simulink library "SUB_L4_Task_10ms_SUB_BRKPEDARB"  (R2018a)
settings: Solver=VariableStepAuto  StartTime=0.0  StopTime=10.0  RelTol=1e-3
libraries: EmE_MBD_Blockset x73, PTC_MBDS_LIB x6, simulink x3
(part 2 of 2)

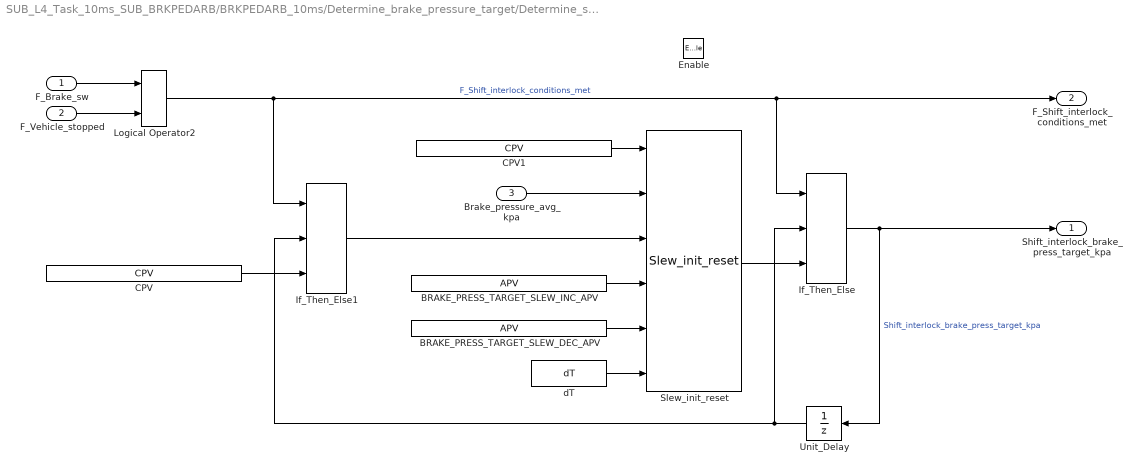
== system SUB_L4_Task_10ms_SUB_BRKPEDARB/BRKPEDARB_10ms/Determine_brake_pressure_target/Determine_shift_interlock_brake_pressure_target ==
  F_Brake_sw : Inport
  F_Vehicle_stopped : Inport  Port=2
  Brake_pressure_avg_kpa : Inport  Port=3
  Enable : EnablePort  StatesWhenEnabling=reset
      settings: AttributesFormatString=States when enabling: %<StatesWhenEnabling>
      settings: CopyFcn=|
      | try
      | L = find_system(get(gcbh,'Parent'),'BlockType','Outport');
      | M = find_system(get(gcbh,'Parent'),'BlockType','EnablePort');
      | N = find_system(get(gcbh,'Parent'),'BlockType','TriggerPort');
      | anyoutports = ~isempty(L);
      | anyenableports = ~isempty(M);
      | anytriggerports = ~isempty(N);
      | sys = get_param(L,'Handle');
      | noutports = length(sys);
      | if (anyoutports),
      | for i = 1:noutports,
      | set(sys{i},'AttributesFormatString','IC: %<InitialOutput>\nDisabled value: %<OutputWhenDisabled>')
      | end;
      | end;
      | catch
      | end;
      | clear i L M N anyoutports anyenableports anytriggerports sys noutports
      settings: DeleteFcn=|
      | try
      | L = find_system(get(gcbh,'Parent'),'BlockType','Outport');
      | M = find_system(get(gcbh,'Parent'),'BlockType','EnablePort');
      | N = find_system(get(gcbh,'Parent'),'BlockType','TriggerPort');
      | anyoutports = ~isempty(L);
      | anyenableports = ~isempty(M);
      | anytriggerports = ~isempty(N);
      | sys = get_param(L,'Handle');
      | noutports = length(sys);
      | if ((anyoutports) && (~anytriggerports)),
      | for i = 1:noutports,
      | set(sys{i},'AttributesFormatString','')
      | end;
      | end;
      | catch
      | end;
      | clear i L M N anyoutports anyenableports anytriggerports sys noutports
      settings: NameChangeFcn=|
      | try
      | L = find_system(get(gcbh,'Parent'),'BlockType','Outport');
      | M = find_system(get(gcbh,'Parent'),'BlockType','EnablePort');
      | N = find_system(get(gcbh,'Parent'),'BlockType','TriggerPort');
      | anyoutports = ~isempty(L);
      | anyenableports = ~isempty(M);
      | anytriggerports = ~isempty(N);
      | sys = get_param(L,'Handle');
      | noutports = length(sys);
      | if (anyoutports),
      | for i = 1:noutports,
      | set(sys{i},'AttributesFormatString','IC: %<InitialOutput>\nDisabled value: %<OutputWhenDisabled>')
      | end;
      | end;
      | catch
      | end
      | clear i L M N anyoutports anyenableports anytriggerports sys noutports
      settings: MoveFcn=|
      | try
      | L = find_system(get(gcbh,'Parent'),'BlockType','Outport');
      | M = find_system(get(gcbh,'Parent'),'BlockType','EnablePort');
      | N = find_system(get(gcbh,'Parent'),'BlockType','TriggerPort');
      | anyoutports = ~isempty(L);
      | anyenableports = ~isempty(M);
      | anytriggerports = ~isempty(N);
      | sys = get_param(L,'Handle');
      | noutports = length(sys);
      | if (anyoutports),
      | for i = 1:noutports,
      | set(sys{i},'AttributesFormatString','IC: %<InitialOutput>\nDisabled value: %<OutputWhenDisabled>')
      | end;
      | end;
      | catch
      | end;
      | clear i L M N anyoutports anyenableports anytriggerports sys noutports
  BRAKE_PRESS_TARGET_SLEW_DEC_APV : EmE_MBD_Blockset/Sources/APV  conval=5000
      settings: SourceProductName=PACCAR EmE MBD Blockset
  BRAKE_PRESS_TARGET_SLEW_INC_APV : EmE_MBD_Blockset/Sources/APV  conval=30
      settings: SourceProductName=PACCAR EmE MBD Blockset
  CPV : EmE_MBD_Blockset/Sources/CPV  conval=865
      settings: SourceProductName=PACCAR EmE MBD Blockset
  CPV1 : EmE_MBD_Blockset/Sources/CPV  conval=false
      settings: SourceProductName=PACCAR EmE MBD Blockset
  If_Then_Else : EmE_MBD_Blockset/Signal Routing/If_Then_Else
      settings: SourceProductName=PACCAR EmE MBD Blockset
  If_Then_Else1 : EmE_MBD_Blockset/Signal Routing/If_Then_Else
      settings: SourceProductName=PACCAR EmE MBD Blockset
  Logical Operator2 : EmE_MBD_Blockset/Logic and Bit Operations/Logical Operator  Operator=AND  Inputs=2
      settings: SourceProductName=PACCAR EmE MBD Blockset
  Slew_init_reset : EmE_MBD_Blockset/Math Operators/Slew_init_reset
      settings: SourceProductName=PACCAR EmE MBD Blockset
  Unit_Delay : UnitDelay  SampleTime=-1
      settings: AttributesFormatString=IC: %<vinit>
  dT : EmE_MBD_Blockset/Sources/dT
      settings: SourceProductName=PACCAR EmE MBD Blockset
  Shift_interlock_brake_press_target_kpa : Outport  OutputWhenDisabled=reset  InitialOutput=0
      settings: AttributesFormatString=IC: %<InitialOutput>\nDisabled value: %<OutputWhenDisabled>
  F_Shift_interlock_conditions_met : Outport  Port=2  OutputWhenDisabled=reset  InitialOutput=false
      settings: AttributesFormatString=IC: %<InitialOutput>\nDisabled value: %<OutputWhenDisabled>
  wires:
  CPV1/1 -> Slew_init_reset/1
  Brake_pressure_avg_kpa/1 -> Slew_init_reset/2
  Logical Operator2/1 -> If_Then_Else/1, F_Shift_interlock_conditions_met/1, If_Then_Else1/1  "F_Shift_interlock_conditions_met"
  BRAKE_PRESS_TARGET_SLEW_INC_APV/1 -> Slew_init_reset/4
  dT/1 -> Slew_init_reset/6
  Slew_init_reset/1 -> If_Then_Else/3
  Unit_Delay/1 -> If_Then_Else/2, If_Then_Else1/2
  If_Then_Else/1 -> Shift_interlock_brake_press_target_kpa/1, Unit_Delay/1  "Shift_interlock_brake_press_target_kpa"
  BRAKE_PRESS_TARGET_SLEW_DEC_APV/1 -> Slew_init_reset/5
  CPV/1 -> If_Then_Else1/3
  F_Vehicle_stopped/1 -> Logical Operator2/2
  F_Brake_sw/1 -> Logical Operator2/1
  If_Then_Else1/1 -> Slew_init_reset/3
